simulink library "mylib"  (R2020a)
settings: Solver=VariableStepAuto  StartTime=0.0  StopTime=10.0  RelTol=1e-3
undefined symbols (not defined in the file): d_du_max_pu, dir_to_bus1, dir_to_bus_0L, dir_to_bus_2, dir_to_line1, dir_to_line_0L, dir_to_line_2, du_max_pu, du_ph_max_pu, Fi_0, Fi_T_H, Fi_T_L, Fi_T_M, I0_calc_0L, I0_comp_H, I0_comp_L, I0_comp_M, I0_max_0L, I2_max_2, I_diff1, I_diff2, I_diff3, I_diff4, I_diff5, I_diff_to, I_hight_CT1_G, I_hight_CT2_G, I_low_CT1, I_low_CT2, I_max1, I_max2, I_max3, I_max4, I_max5, I_min_sec_CT1, I_min_sec_CT2, I_unb, Iph_max_0L, Iph_max_2, jmp_in_zone, jmp_in_zone_0L, jmp_in_zone_2, K_dop, max_min1, only_K1_0L, only_K1_2, only_K2_0L, only_K2_2, only_K3_0L, only_K3_2, P_ctl_0, PQ_Fi_ctl_0, Q_ctl_0, S_set_0, set, set1, T_fast, T_I_ctl, T_off, T_on ... (+15)
libraries: $bdroot x184, powerlib_meascontrol x97
(part 13 of 14)

== system mylib/Inverse time-delay/IEC Inverse time-delay/Equation IEC/Zero_check ==
  in : Inport
  Constant : Constant  Value=0
  Constant1 : Constant  Value=0.000001
  Relational Operator : RelationalOperator  Operator===  OutDataTypeStr=boolean  RndMeth=Simplest
  Switch : Switch  Criteria=u2 > Threshold
  out : Outport
  wires:
  in/1 -> Switch/3, Relational Operator/1
  Constant/1 -> Relational Operator/2
  Relational Operator/1 -> Switch/2
  Constant1/1 -> Switch/1
  Switch/1 -> out/1

== system mylib/Inverse time-delay/IEC Inverse time-delay/Equation IEC/Zero_check1 ==
  in : Inport
  Constant : Constant  Value=0
  Constant1 : Constant  Value=0.000001
  Relational Operator : RelationalOperator  Operator===  OutDataTypeStr=boolean  RndMeth=Simplest
  Switch : Switch  Criteria=u2 > Threshold
  out : Outport
  wires:
  in/1 -> Switch/3, Relational Operator/1
  Constant/1 -> Relational Operator/2
  Relational Operator/1 -> Switch/2
  Constant1/1 -> Switch/1
  Switch/1 -> out/1

== system mylib/Inverse time-delay/IEC Inverse time-delay inductive disk relay/Equation IEC_idr/Zero_check ==
  in : Inport
  Constant : Constant  Value=0
  Constant1 : Constant  Value=0.000001
  Relational Operator : RelationalOperator  Operator===  OutDataTypeStr=boolean  RndMeth=Simplest
  Switch : Switch  Criteria=u2 > Threshold
  out : Outport
  wires:
  in/1 -> Switch/3, Relational Operator/1
  Constant/1 -> Relational Operator/2
  Relational Operator/1 -> Switch/2
  Constant1/1 -> Switch/1
  Switch/1 -> out/1

== system mylib/Inverse time-delay/IEC Inverse time-delay inductive disk relay/Equation IEC_idr/Zero_check1 ==
  in : Inport
  Constant : Constant  Value=0
  Constant1 : Constant  Value=0.000001
  Relational Operator : RelationalOperator  Operator===  OutDataTypeStr=boolean  RndMeth=Simplest
  Switch : Switch  Criteria=u2 > Threshold
  out : Outport
  wires:
  in/1 -> Switch/3, Relational Operator/1
  Constant/1 -> Relational Operator/2
  Relational Operator/1 -> Switch/2
  Constant1/1 -> Switch/1
  Switch/1 -> out/1

== system mylib/st_inverse/Inverse time-delay/ANSI Inverse time-delay/Equation ANSI ==
  B : Inport
  I : Inport  Port=2
  Ip : Inport  Port=3
  A : Inport  Port=4
  C : Inport  Port=5
  D : Inport  Port=6
  Add : Sum  Inputs=+-
  Add1 : Sum
  Constant18 : Constant  Value=20
  Constant3 : Constant
  Divide : Product  Inputs=*/
  Divide1 : Product  Inputs=*/
  Divide3 : Product  Inputs=**
  Math Function : Math  Operator=pow  SaturateOnIntegerOverflow=on
  Relational Operator : RelationalOperator  OutDataTypeStr=boolean  RndMeth=Simplest
  Switch : Switch  Criteria=u2 > Threshold
  Zero_check : Subsystem
  Zero_check1 : Subsystem
  td : Outport
  wires:
  I/1 -> Divide/1
  B/1 -> Divide1/1
  D/1 -> Divide3/2
  Divide3/1 -> td/1
  Ip/1 -> Zero_check/1(in)
  Zero_check/1(out) -> Divide/2
  Add/1 -> Zero_check1/1(in)
  Zero_check1/1(out) -> Divide1/2
  Constant3/1 -> Add/2
  Divide1/1 -> Add1/1
  Add1/1 -> Divide3/1
  C/1 -> Add1/2
  Divide/1 -> Switch/3, Relational Operator/1
  Constant18/1 -> Switch/1, Relational Operator/2
  Relational Operator/1 -> Switch/2
  Switch/1 -> Math Function/1
  A/1 -> Math Function/2
  Math Function/1 -> Add/1

== system mylib/st_inverse/Inverse time-delay/ANSI Inverse time-delay/Сoefficient_1 ==
  A_in : Inport
  B_in : Inport  Port=2
  C_in : Inport  Port=3
  N : Inport  Port=4
  Constant1 : Constant  Value=0.17966
  Constant3 : Constant  Value=2.0938
  Constant6 : Constant  Value=8.9341
  Switch : Switch  Criteria=u2 > Threshold
  Switch1 : Switch  Criteria=u2 > Threshold
  Switch2 : Switch  Criteria=u2 > Threshold
  A_out : Outport
  B_out : Outport  Port=2
  C_out : Outport  Port=3
  wires:
  Switch1/1 -> B_out/1
  Constant3/1 -> Switch/1
  Constant6/1 -> Switch1/1
  Switch/1 -> A_out/1
  N/1 -> Switch2/2, Switch/2, Switch1/2
  A_in/1 -> Switch/3
  B_in/1 -> Switch1/3
  C_in/1 -> Switch2/3
  Constant1/1 -> Switch2/1
  Switch2/1 -> C_out/1

== system mylib/st_inverse/Inverse time-delay/ANSI Inverse time-delay/Сoefficient_2 ==
  A_in : Inport
  B_in : Inport  Port=2
  C_in : Inport  Port=3
  N : Inport  Port=4
  Constant1 : Constant  Value=0.03393
  Constant3 : Constant  Value=1.2969
  Constant6 : Constant  Value=0.2663
  Switch : Switch  Criteria=u2 > Threshold
  Switch1 : Switch  Criteria=u2 > Threshold
  Switch2 : Switch  Criteria=u2 > Threshold
  A_out : Outport
  B_out : Outport  Port=2
  C_out : Outport  Port=3
  wires:
  Switch1/1 -> B_out/1
  Constant3/1 -> Switch/1
  Constant6/1 -> Switch1/1
  Switch/1 -> A_out/1
  N/1 -> Switch2/2, Switch/2, Switch1/2
  A_in/1 -> Switch/3
  B_in/1 -> Switch1/3
  C_in/1 -> Switch2/3
  Constant1/1 -> Switch2/1
  Switch2/1 -> C_out/1

== system mylib/st_inverse/Inverse time-delay/ANSI Inverse time-delay/Сoefficient_3 ==
  A_in : Inport
  B_in : Inport  Port=2
  C_in : Inport  Port=3
  N : Inport  Port=4
  Constant1 : Constant  Value=2.18592
  Constant3 : Constant
  Constant6 : Constant  Value=5.6143
  Switch : Switch  Criteria=u2 > Threshold
  Switch1 : Switch  Criteria=u2 > Threshold
  Switch2 : Switch  Criteria=u2 > Threshold
  A_out : Outport
  B_out : Outport  Port=2
  C_out : Outport  Port=3
  wires:
  Switch1/1 -> B_out/1
  Constant3/1 -> Switch/1
  Constant6/1 -> Switch1/1
  Switch/1 -> A_out/1
  N/1 -> Switch2/2, Switch/2, Switch1/2
  A_in/1 -> Switch/3
  B_in/1 -> Switch1/3
  C_in/1 -> Switch2/3
  Constant1/1 -> Switch2/1
  Switch2/1 -> C_out/1

== system mylib/st_inverse/Inverse time-delay/ANSI Inverse time-delay/Сoefficient_4 ==
  A_in : Inport
  B_in : Inport  Port=2
  C_in : Inport  Port=3
  N : Inport  Port=4
  Constant1 : Constant  Value=0.0228
  Constant3 : Constant  Value=0.02
  Constant6 : Constant  Value=0.0103
  Switch : Switch  Criteria=u2 > Threshold
  Switch1 : Switch  Criteria=u2 > Threshold
  Switch2 : Switch  Criteria=u2 > Threshold
  A_out : Outport
  B_out : Outport  Port=2
  C_out : Outport  Port=3
  wires:
  Switch1/1 -> B_out/1
  Constant3/1 -> Switch/1
  Constant6/1 -> Switch1/1
  Switch/1 -> A_out/1
  N/1 -> Switch2/2, Switch/2, Switch1/2
  A_in/1 -> Switch/3
  B_in/1 -> Switch1/3
  C_in/1 -> Switch2/3
  Constant1/1 -> Switch2/1
  Switch2/1 -> C_out/1

== system mylib/st_inverse/Inverse time-delay/ANSI Inverse time-delay/Сoefficient_5 ==
  A_in : Inport
  B_in : Inport  Port=2
  C_in : Inport  Port=3
  N : Inport  Port=4
  Constant1 : Constant  Value=0.0982
  Constant3 : Constant  Value=2
  Constant6 : Constant  Value=3.922
  Switch : Switch  Criteria=u2 > Threshold
  Switch1 : Switch  Criteria=u2 > Threshold
  Switch2 : Switch  Criteria=u2 > Threshold
  A_out : Outport
  B_out : Outport  Port=2
  C_out : Outport  Port=3
  wires:
  Switch1/1 -> B_out/1
  Constant3/1 -> Switch/1
  Constant6/1 -> Switch1/1
  Switch/1 -> A_out/1
  N/1 -> Switch2/2, Switch/2, Switch1/2
  A_in/1 -> Switch/3
  B_in/1 -> Switch1/3
  C_in/1 -> Switch2/3
  Constant1/1 -> Switch2/1
  Switch2/1 -> C_out/1

== system mylib/st_inverse/Inverse time-delay/ANSI Inverse time-delay/Сoefficient_6 ==
  A_in : Inport
  B_in : Inport  Port=2
  C_in : Inport  Port=3
  N : Inport  Port=4
  Constant1 : Constant  Value=0.02434
  Constant3 : Constant  Value=2
  Constant6 : Constant  Value=5.64
  Switch : Switch  Criteria=u2 > Threshold
  Switch1 : Switch  Criteria=u2 > Threshold
  Switch2 : Switch  Criteria=u2 > Threshold
  A_out : Outport
  B_out : Outport  Port=2
  C_out : Outport  Port=3
  wires:
  Switch1/1 -> B_out/1
  Constant3/1 -> Switch/1
  Constant6/1 -> Switch1/1
  Switch/1 -> A_out/1
  N/1 -> Switch2/2, Switch/2, Switch1/2
  A_in/1 -> Switch/3
  B_in/1 -> Switch1/3
  C_in/1 -> Switch2/3
  Constant1/1 -> Switch2/1
  Switch2/1 -> C_out/1

== system mylib/st_inverse/Inverse time-delay/ANSI Inverse time-delay/Сoefficient_7 ==
  A_in : Inport
  B_in : Inport  Port=2
  C_in : Inport  Port=3
  N : Inport  Port=4
  Constant1 : Constant  Value=0.21359
  Constant3 : Constant  Value=1.5825
  Constant6 : Constant  Value=0.4797
  Switch : Switch  Criteria=u2 > Threshold
  Switch1 : Switch  Criteria=u2 > Threshold
  Switch2 : Switch  Criteria=u2 > Threshold
  A_out : Outport
  B_out : Outport  Port=2
  C_out : Outport  Port=3
  wires:
  Switch1/1 -> B_out/1
  Constant3/1 -> Switch/1
  Constant6/1 -> Switch1/1
  Switch/1 -> A_out/1
  N/1 -> Switch2/2, Switch/2, Switch1/2
  A_in/1 -> Switch/3
  B_in/1 -> Switch1/3
  C_in/1 -> Switch2/3
  Constant1/1 -> Switch2/1
  Switch2/1 -> C_out/1

== system mylib/st_inverse/Inverse time-delay/ANSI Inverse time-delay/Сoefficient_8 User ==
  A_in : Inport
  B_in : Inport  Port=2
  C_in : Inport  Port=3
  N : Inport  Port=4
  Au : Inport  Port=5
  Bu : Inport  Port=6
  Cu : Inport  Port=7
  Switch : Switch  Criteria=u2 > Threshold
  Switch1 : Switch  Criteria=u2 > Threshold
  Switch2 : Switch  Criteria=u2 > Threshold
  B_out : Outport
  A_out : Outport  Port=2
  C_out : Outport  Port=3
  wires:
  Switch1/1 -> B_out/1
  Au/1 -> Switch/1
  Bu/1 -> Switch1/1
  Switch/1 -> A_out/1
  N/1 -> Switch2/2, Switch/2, Switch1/2
  A_in/1 -> Switch/3
  B_in/1 -> Switch1/3
  C_in/1 -> Switch2/3
  Cu/1 -> Switch2/1
  Switch2/1 -> C_out/1

== system mylib/st_inverse/Inverse time-delay/ANSI Inverse time-delay inductive disk relay/Equation ANSI_idr ==
  B : Inport
  I : Inport  Port=2
  Ip : Inport  Port=3
  A : Inport  Port=4
  C : Inport  Port=5
  D : Inport  Port=6
  Add : Sum  Inputs=+-
  Add1 : Sum
  Constant3 : Constant
  Divide : Product  Inputs=*/
  Divide1 : Product  Inputs=*/
  Divide3 : Product  Inputs=**
  Math Function : Math  Operator=pow  SaturateOnIntegerOverflow=on
  Zero_check : Subsystem
  Zero_check1 : Subsystem
  td : Outport
  wires:
  I/1 -> Divide/1
  B/1 -> Divide1/1
  D/1 -> Divide3/2
  Divide3/1 -> td/1
  Divide/1 -> Math Function/1
  A/1 -> Math Function/2
  Ip/1 -> Zero_check/1(in)
  Zero_check/1(out) -> Divide/2
  Add/1 -> Zero_check1/1(in)
  Zero_check1/1(out) -> Divide1/2
  Constant3/1 -> Add/1
  Divide1/1 -> Add1/1
  Add1/1 -> Divide3/1
  C/1 -> Add1/2
  Math Function/1 -> Add/2

== system mylib/st_inverse/Inverse time-delay/ANSI Inverse time-delay inductive disk relay/Сoefficient_1 ==
  A_in : Inport
  B_in : Inport  Port=2
  C_in : Inport  Port=3
  N : Inport  Port=4
  Constant1 : Constant  Value=0
  Constant3 : Constant  Value=2.0938
  Constant6 : Constant  Value=8.8
  Switch : Switch  Criteria=u2 > Threshold
  Switch1 : Switch  Criteria=u2 > Threshold
  Switch2 : Switch  Criteria=u2 > Threshold
  A_out : Outport
  B_out : Outport  Port=2
  C_out : Outport  Port=3
  wires:
  Switch1/1 -> B_out/1
  Constant3/1 -> Switch/1
  Constant6/1 -> Switch1/1
  Switch/1 -> A_out/1
  N/1 -> Switch2/2, Switch/2, Switch1/2
  A_in/1 -> Switch/3
  B_in/1 -> Switch1/3
  C_in/1 -> Switch2/3
  Constant1/1 -> Switch2/1
  Switch2/1 -> C_out/1

== system mylib/st_inverse/Inverse time-delay/ANSI Inverse time-delay inductive disk relay/Сoefficient_2 ==
  A_in : Inport
  B_in : Inport  Port=2
  C_in : Inport  Port=3
  N : Inport  Port=4
  Constant1 : Constant  Value=0
  Constant3 : Constant  Value=1.2969
  Constant6 : Constant  Value=0.831
  Switch : Switch  Criteria=u2 > Threshold
  Switch1 : Switch  Criteria=u2 > Threshold
  Switch2 : Switch  Criteria=u2 > Threshold
  A_out : Outport
  B_out : Outport  Port=2
  C_out : Outport  Port=3
  wires:
  Switch1/1 -> B_out/1
  Constant3/1 -> Switch/1
  Constant6/1 -> Switch1/1
  Switch/1 -> A_out/1
  N/1 -> Switch2/2, Switch/2, Switch1/2
  A_in/1 -> Switch/3
  B_in/1 -> Switch1/3
  C_in/1 -> Switch2/3
  Constant1/1 -> Switch2/1
  Switch2/1 -> C_out/1

== system mylib/st_inverse/Inverse time-delay/ANSI Inverse time-delay inductive disk relay/Сoefficient_3 ==
  A_in : Inport
  B_in : Inport  Port=2
  C_in : Inport  Port=3
  N : Inport  Port=4
  Constant1 : Constant  Value=0
  Constant3 : Constant
  Constant6 : Constant  Value=12.9
  Switch : Switch  Criteria=u2 > Threshold
  Switch1 : Switch  Criteria=u2 > Threshold
  Switch2 : Switch  Criteria=u2 > Threshold
  A_out : Outport
  B_out : Outport  Port=2
  C_out : Outport  Port=3
  wires:
  Switch1/1 -> B_out/1
  Constant3/1 -> Switch/1
  Constant6/1 -> Switch1/1
  Switch/1 -> A_out/1
  N/1 -> Switch2/2, Switch/2, Switch1/2
  A_in/1 -> Switch/3
  B_in/1 -> Switch1/3
  C_in/1 -> Switch2/3
  Constant1/1 -> Switch2/1
  Switch2/1 -> C_out/1

== system mylib/st_inverse/Inverse time-delay/ANSI Inverse time-delay inductive disk relay/Сoefficient_4 ==
  A_in : Inport
  B_in : Inport  Port=2
  C_in : Inport  Port=3
  N : Inport  Port=4
  Constant1 : Constant  Value=0
  Constant3 : Constant  Value=2
  Constant6 : Constant  Value=0.97
  Switch : Switch  Criteria=u2 > Threshold
  Switch1 : Switch  Criteria=u2 > Threshold
  Switch2 : Switch  Criteria=u2 > Threshold
  A_out : Outport
  B_out : Outport  Port=2
  C_out : Outport  Port=3
  wires:
  Switch1/1 -> B_out/1
  Constant3/1 -> Switch/1
  Constant6/1 -> Switch1/1
  Switch/1 -> A_out/1
  N/1 -> Switch2/2, Switch/2, Switch1/2
  A_in/1 -> Switch/3
  B_in/1 -> Switch1/3
  C_in/1 -> Switch2/3
  Constant1/1 -> Switch2/1
  Switch2/1 -> C_out/1

== system mylib/st_inverse/Inverse time-delay/ANSI Inverse time-delay inductive disk relay/Сoefficient_5 ==
  A_in : Inport
  B_in : Inport  Port=2
  C_in : Inport  Port=3
  N : Inport  Port=4
  Constant1 : Constant  Value=0
  Constant3 : Constant  Value=2
  Constant6 : Constant  Value=4.32
  Switch : Switch  Criteria=u2 > Threshold
  Switch1 : Switch  Criteria=u2 > Threshold
  Switch2 : Switch  Criteria=u2 > Threshold
  A_out : Outport
  B_out : Outport  Port=2
  C_out : Outport  Port=3
  wires:
  Switch1/1 -> B_out/1
  Constant3/1 -> Switch/1
  Constant6/1 -> Switch1/1
  Switch/1 -> A_out/1
  N/1 -> Switch2/2, Switch/2, Switch1/2
  A_in/1 -> Switch/3
  B_in/1 -> Switch1/3
  C_in/1 -> Switch2/3
  Constant1/1 -> Switch2/1
  Switch2/1 -> C_out/1

== system mylib/st_inverse/Inverse time-delay/ANSI Inverse time-delay inductive disk relay/Сoefficient_6 ==
  A_in : Inport
  B_in : Inport  Port=2
  C_in : Inport  Port=3
  N : Inport  Port=4
  Constant1 : Constant  Value=0
  Constant3 : Constant  Value=2
  Constant6 : Constant  Value=5.82
  Switch : Switch  Criteria=u2 > Threshold
  Switch1 : Switch  Criteria=u2 > Threshold
  Switch2 : Switch  Criteria=u2 > Threshold
  A_out : Outport
  B_out : Outport  Port=2
  C_out : Outport  Port=3
  wires:
  Switch1/1 -> B_out/1
  Constant3/1 -> Switch/1
  Constant6/1 -> Switch1/1
  Switch/1 -> A_out/1
  N/1 -> Switch2/2, Switch/2, Switch1/2
  A_in/1 -> Switch/3
  B_in/1 -> Switch1/3
  C_in/1 -> Switch2/3
  Constant1/1 -> Switch2/1
  Switch2/1 -> C_out/1

== system mylib/st_inverse/Inverse time-delay/ANSI Inverse time-delay inductive disk relay/Сoefficient_7 ==
  A_in : Inport
  B_in : Inport  Port=2
  C_in : Inport  Port=3
  N : Inport  Port=4
  Constant1 : Constant  Value=0.21359
  Constant3 : Constant  Value=1.5625
  Constant6 : Constant  Value=1.0394
  Switch : Switch  Criteria=u2 > Threshold
  Switch1 : Switch  Criteria=u2 > Threshold
  Switch2 : Switch  Criteria=u2 > Threshold
  A_out : Outport
  B_out : Outport  Port=2
  C_out : Outport  Port=3
  wires:
  Switch1/1 -> B_out/1
  Constant3/1 -> Switch/1
  Constant6/1 -> Switch1/1
  Switch/1 -> A_out/1
  N/1 -> Switch2/2, Switch/2, Switch1/2
  A_in/1 -> Switch/3
  B_in/1 -> Switch1/3
  C_in/1 -> Switch2/3
  Constant1/1 -> Switch2/1
  Switch2/1 -> C_out/1

== system mylib/st_inverse/Inverse time-delay/ANSI Inverse time-delay inductive disk relay/Сoefficient_8 User ==
  A_in : Inport
  B_in : Inport  Port=2
  C_in : Inport  Port=3
  N : Inport  Port=4
  Au : Inport  Port=5
  Bu : Inport  Port=6
  Cu : Inport  Port=7
  Switch : Switch  Criteria=u2 > Threshold
  Switch1 : Switch  Criteria=u2 > Threshold
  Switch2 : Switch  Criteria=u2 > Threshold
  B_out : Outport
  A_out : Outport  Port=2
  C_out : Outport  Port=3
  wires:
  Switch1/1 -> B_out/1
  Au/1 -> Switch/1
  Bu/1 -> Switch1/1
  Switch/1 -> A_out/1
  N/1 -> Switch2/2, Switch/2, Switch1/2
  A_in/1 -> Switch/3
  B_in/1 -> Switch1/3
  C_in/1 -> Switch2/3
  Cu/1 -> Switch2/1
  Switch2/1 -> C_out/1

== system mylib/st_inverse/Inverse time-delay/IEC Inverse time-delay/Equation IEC ==
  k : Inport
  I : Inport  Port=2
  a : Inport  Port=3
  Ip : Inport  Port=4
  Tb : Inport  Port=5
  Add : Sum  Inputs=+-
  Constant18 : Constant  Value=20
  Constant3 : Constant
  Divide : Product  Inputs=*/
  Divide1 : Product  Inputs=*/
  Divide2 : Product  Inputs=*/
  Divide3 : Product  Inputs=**
  Math Function : Math  Operator=pow  SaturateOnIntegerOverflow=on
  Relational Operator : RelationalOperator  OutDataTypeStr=boolean  RndMeth=Simplest
  Switch : Switch  Criteria=u2 > Threshold
  Zero_check : Subsystem
  Zero_check1 : Subsystem
  td : Outport
  wires:
  I/1 -> Divide/1, Divide2/1
  Math Function/1 -> Add/1
  Constant3/1 -> Add/2
  k/1 -> Divide1/1
  Divide1/1 -> Divide3/1
  Tb/1 -> Divide3/2
  Divide3/1 -> td/1
  a/1 -> Math Function/2
  Ip/1 -> Zero_check/1(in)
  Zero_check/1(out) -> Divide2/2, Divide/2
  Add/1 -> Zero_check1/1(in)
  Zero_check1/1(out) -> Divide1/2
  Divide2/1 -> Relational Operator/1
  Constant18/1 -> Switch/1, Relational Operator/2
  Relational Operator/1 -> Switch/2
  Divide/1 -> Switch/3
  Switch/1 -> Math Function/1

== system mylib/st_inverse/Inverse time-delay/IEC Inverse time-delay/Сoefficient_1 ==
  k_in : Inport
  a_in : Inport  Port=2
  N : Inport  Port=3
  Constant3 : Constant  Value=0.14
  Constant6 : Constant  Value=0.02
  Switch : Switch  Criteria=u2 > Threshold
  Switch1 : Switch  Criteria=u2 > Threshold
  k_out : Outport
  a_out : Outport  Port=2
  wires:
  Switch1/1 -> a_out/1
  Constant3/1 -> Switch/1
  Constant6/1 -> Switch1/1
  Switch/1 -> k_out/1
  N/1 -> Switch/2, Switch1/2
  k_in/1 -> Switch/3
  a_in/1 -> Switch1/3

== system mylib/st_inverse/Inverse time-delay/IEC Inverse time-delay/Сoefficient_2 ==
  k_in : Inport
  a_in : Inport  Port=2
  N : Inport  Port=3
  Constant3 : Constant  Value=13.5
  Constant6 : Constant
  Switch : Switch  Criteria=u2 > Threshold
  Switch1 : Switch  Criteria=u2 > Threshold
  k_out : Outport
  a_out : Outport  Port=2
  wires:
  Switch1/1 -> a_out/1
  Constant3/1 -> Switch/1
  Constant6/1 -> Switch1/1
  Switch/1 -> k_out/1
  N/1 -> Switch/2, Switch1/2
  k_in/1 -> Switch/3
  a_in/1 -> Switch1/3

== system mylib/st_inverse/Inverse time-delay/IEC Inverse time-delay/Сoefficient_3 ==
  k_in : Inport
  a_in : Inport  Port=2
  N : Inport  Port=3
  Constant3 : Constant  Value=120
  Constant6 : Constant
  Switch : Switch  Criteria=u2 > Threshold
  Switch1 : Switch  Criteria=u2 > Threshold
  k_out : Outport
  a_out : Outport  Port=2
  wires:
  Switch1/1 -> a_out/1
  Constant3/1 -> Switch/1
  Constant6/1 -> Switch1/1
  Switch/1 -> k_out/1
  N/1 -> Switch/2, Switch1/2
  k_in/1 -> Switch/3
  a_in/1 -> Switch1/3

== system mylib/st_inverse/Inverse time-delay/IEC Inverse time-delay/Сoefficient_4 ==
  k_in : Inport
  a_in : Inport  Port=2
  N : Inport  Port=3
  Constant3 : Constant  Value=80
  Constant6 : Constant  Value=2
  Switch : Switch  Criteria=u2 > Threshold
  Switch1 : Switch  Criteria=u2 > Threshold
  k_out : Outport
  a_out : Outport  Port=2
  wires:
  Switch1/1 -> a_out/1
  Constant3/1 -> Switch/1
  Constant6/1 -> Switch1/1
  Switch/1 -> k_out/1
  N/1 -> Switch/2, Switch1/2
  k_in/1 -> Switch/3
  a_in/1 -> Switch1/3

== system mylib/st_inverse/Inverse time-delay/IEC Inverse time-delay/Сoefficient_5 User ==
  k : Inport
  a : Inport  Port=2
  N : Inport  Port=3
  k_u : Inport  Port=4
  a_u : Inport  Port=5
  Switch : Switch  Criteria=u2 > Threshold
  Switch1 : Switch  Criteria=u2 > Threshold
  k_out : Outport
  a_out : Outport  Port=2
  wires:
  Switch1/1 -> a_out/1
  k_u/1 -> Switch/1
  a_u/1 -> Switch1/1
  Switch/1 -> k_out/1
  N/1 -> Switch/2, Switch1/2
  k/1 -> Switch/3
  a/1 -> Switch1/3

== system mylib/st_inverse/Inverse time-delay/IEC Inverse time-delay inductive disk relay/Equation IEC_idr ==
  k : Inport
  I : Inport  Port=2
  a : Inport  Port=3
  Ip : Inport  Port=4
  Tb : Inport  Port=5
  Add : Sum  Inputs=+-
  Constant3 : Constant
  Divide : Product  Inputs=*/
  Divide1 : Product  Inputs=*/
  Divide3 : Product  Inputs=**
  Math Function : Math  Operator=pow  SaturateOnIntegerOverflow=on
  Zero_check : Subsystem
  Zero_check1 : Subsystem
  td : Outport
  wires:
  I/1 -> Divide/1
  k/1 -> Divide1/1
  Divide1/1 -> Divide3/1
  Tb/1 -> Divide3/2
  Divide3/1 -> td/1
  Divide/1 -> Math Function/1
  a/1 -> Math Function/2
  Ip/1 -> Zero_check/1(in)
  Zero_check/1(out) -> Divide/2
  Add/1 -> Zero_check1/1(in)
  Zero_check1/1(out) -> Divide1/2
  Math Function/1 -> Add/2
  Constant3/1 -> Add/1

== system mylib/st_inverse/Inverse time-delay/IEC Inverse time-delay inductive disk relay/Сoefficient_1 ==
  k_in : Inport
  a_in : Inport  Port=2
  N : Inport  Port=3
  Constant3 : Constant  Value=9.7
  Constant6 : Constant  Value=2
  Switch : Switch  Criteria=u2 > Threshold
  Switch1 : Switch  Criteria=u2 > Threshold
  k_out : Outport
  a_out : Outport  Port=2
  wires:
  Switch1/1 -> a_out/1
  Constant3/1 -> Switch/1
  Constant6/1 -> Switch1/1
  Switch/1 -> k_out/1
  N/1 -> Switch/2, Switch1/2
  k_in/1 -> Switch/3
  a_in/1 -> Switch1/3

== system mylib/st_inverse/Inverse time-delay/IEC Inverse time-delay inductive disk relay/Сoefficient_2 ==
  k_in : Inport
  a_in : Inport  Port=2
  N : Inport  Port=3
  Constant3 : Constant  Value=43.2
  Constant6 : Constant  Value=2
  Switch : Switch  Criteria=u2 > Threshold
  Switch1 : Switch  Criteria=u2 > Threshold
  k_out : Outport
  a_out : Outport  Port=2
  wires:
  Switch1/1 -> a_out/1
  Constant3/1 -> Switch/1
  Constant6/1 -> Switch1/1
  Switch/1 -> k_out/1
  N/1 -> Switch/2, Switch1/2
  k_in/1 -> Switch/3
  a_in/1 -> Switch1/3

== system mylib/st_inverse/Inverse time-delay/IEC Inverse time-delay inductive disk relay/Сoefficient_3 ==
  k_in : Inport
  a_in : Inport  Port=2
  N : Inport  Port=3
  Constant3 : Constant  Value=58.2
  Constant6 : Constant  Value=2
  Switch : Switch  Criteria=u2 > Threshold
  Switch1 : Switch  Criteria=u2 > Threshold
  k_out : Outport
  a_out : Outport  Port=2
  wires:
  Switch1/1 -> a_out/1
  Constant3/1 -> Switch/1
  Constant6/1 -> Switch1/1
  Switch/1 -> k_out/1
  N/1 -> Switch/2, Switch1/2
  k_in/1 -> Switch/3
  a_in/1 -> Switch1/3

== system mylib/st_inverse/Inverse time-delay/IEC Inverse time-delay inductive disk relay/Сoefficient_4 ==
  k_in : Inport
  a_in : Inport  Port=2
  N : Inport  Port=3
  Constant3 : Constant  Value=80
  Constant6 : Constant  Value=2
  Switch : Switch  Criteria=u2 > Threshold
  Switch1 : Switch  Criteria=u2 > Threshold
  k_out : Outport
  a_out : Outport  Port=2
  wires:
  Switch1/1 -> a_out/1
  Constant3/1 -> Switch/1
  Constant6/1 -> Switch1/1
  Switch/1 -> k_out/1
  N/1 -> Switch/2, Switch1/2
  k_in/1 -> Switch/3
  a_in/1 -> Switch1/3

== system mylib/st_inverse/Inverse time-delay/IEC Inverse time-delay inductive disk relay/Сoefficient_5 User ==
  k : Inport
  a : Inport  Port=2
  N : Inport  Port=3
  k_u : Inport  Port=4
  a_u : Inport  Port=5
  Switch : Switch  Criteria=u2 > Threshold
  Switch1 : Switch  Criteria=u2 > Threshold
  k_out : Outport
  a_out : Outport  Port=2
  wires:
  Switch1/1 -> a_out/1
  k_u/1 -> Switch/1
  a_u/1 -> Switch1/1
  Switch/1 -> k_out/1
  N/1 -> Switch/2, Switch1/2
  k/1 -> Switch/3
  a/1 -> Switch1/3

== system mylib/278_dzt_v1/diff_brake/calc_brake_Ia/cut_brake_1/ADD_B ==
  Y1 : Inport
  X2 : Inport  Port=2
  Y2 : Inport  Port=3
  X1 : Inport  Port=4
  1 : Product
  2 : Sum  Inputs=+-
  3 : Product  Inputs=*/  RndMeth=Zero  SaturateOnIntegerOverflow=on
  4 : Product
  5 : Sum  Inputs=+-
  out : Outport
  wires:
  3/1 -> out/1
  4/1 -> 5/2
  Y2/1 -> 4/1
  2/1 -> 3/2
  5/1 -> 3/1
  1/1 -> 5/1
  X2/1 -> 2/1, 1/2
  X1/1 -> 4/2, 2/2
  Y1/1 -> 1/1

== system mylib/278_dzt_v1/diff_brake/calc_brake_Ia/cut_brake_1/ADD_K ==
  Y2 : Inport
  Y1 : Inport  Port=2
  X2 : Inport  Port=3
  X1 : Inport  Port=4
  1 : Sum  Inputs=+-
  2 : Sum  Inputs=+-
  3 : Product  Inputs=*/  RndMeth=Zero  SaturateOnIntegerOverflow=on
  out : Outport
  wires:
  Y1/1 -> 1/2
  Y2/1 -> 1/1
  X1/1 -> 2/2
  X2/1 -> 2/1
  3/1 -> out/1
  2/1 -> 3/2
  1/1 -> 3/1

== system mylib/278_dzt_v1/diff_brake/calc_brake_Ia/cut_brake_1/z_ch ==
  in1 : Inport
  in2 : Inport  Port=2
  1 : RelationalOperator  Operator===  OutDataTypeStr=boolean  RndMeth=Simplest
  2 : RelationalOperator  Operator===  OutDataTypeStr=boolean  RndMeth=Simplest
  3 : Logic  AllPortsSameDT=off  OutDataTypeStr=boolean
  36 : Constant  Value=0
  out : Outport
  wires:
  3/1 -> out/1
  2/1 -> 3/2
  1/1 -> 3/1
  36/1 -> 2/2, 1/2
  in2/1 -> 2/1
  in1/1 -> 1/1

== system mylib/278_dzt_v1/diff_brake/calc_brake_Ia/cut_brake_1/z_ch1 ==
  in1 : Inport
  in2 : Inport  Port=2
  1 : RelationalOperator  Operator===  OutDataTypeStr=boolean  RndMeth=Simplest
  2 : RelationalOperator  Operator===  OutDataTypeStr=boolean  RndMeth=Simplest
  3 : Logic  AllPortsSameDT=off  OutDataTypeStr=boolean
  36 : Constant  Value=0
  out : Outport
  wires:
  3/1 -> out/1
  2/1 -> 3/2
  1/1 -> 3/1
  36/1 -> 2/2, 1/2
  in2/1 -> 2/1
  in1/1 -> 1/1

== system mylib/278_dzt_v1/diff_brake/calc_brake_Ia/cut_brake_1/z_ch2 ==
  in1 : Inport
  in2 : Inport  Port=2
  1 : RelationalOperator  Operator===  OutDataTypeStr=boolean  RndMeth=Simplest
  2 : RelationalOperator  Operator===  OutDataTypeStr=boolean  RndMeth=Simplest
  3 : Logic  AllPortsSameDT=off  OutDataTypeStr=boolean
  36 : Constant  Value=0
  out : Outport
  wires:
  3/1 -> out/1
  2/1 -> 3/2
  1/1 -> 3/1
  36/1 -> 2/2, 1/2
  in2/1 -> 2/1
  in1/1 -> 1/1

== system mylib/278_dzt_v1/diff_brake/calc_brake_Ia/cut_brake_2/ADD_B ==
  Y1 : Inport
  X2 : Inport  Port=2
  Y2 : Inport  Port=3
  X1 : Inport  Port=4
  1 : Product
  2 : Sum  Inputs=+-
  3 : Product  Inputs=*/  RndMeth=Zero  SaturateOnIntegerOverflow=on
  4 : Product
  5 : Sum  Inputs=+-
  out : Outport
  wires:
  3/1 -> out/1
  4/1 -> 5/2
  Y2/1 -> 4/1
  2/1 -> 3/2
  5/1 -> 3/1
  1/1 -> 5/1
  X2/1 -> 2/1, 1/2
  X1/1 -> 4/2, 2/2
  Y1/1 -> 1/1

== system mylib/278_dzt_v1/diff_brake/calc_brake_Ia/cut_brake_2/ADD_K ==
  Y2 : Inport
  Y1 : Inport  Port=2
  X2 : Inport  Port=3
  X1 : Inport  Port=4
  1 : Sum  Inputs=+-
  2 : Sum  Inputs=+-
  3 : Product  Inputs=*/  RndMeth=Zero  SaturateOnIntegerOverflow=on
  out : Outport
  wires:
  Y1/1 -> 1/2
  Y2/1 -> 1/1
  X1/1 -> 2/2
  X2/1 -> 2/1
  3/1 -> out/1
  2/1 -> 3/2
  1/1 -> 3/1

== system mylib/278_dzt_v1/diff_brake/calc_brake_Ia/cut_brake_2/z_ch ==
  in1 : Inport
  in2 : Inport  Port=2
  1 : RelationalOperator  Operator===  OutDataTypeStr=boolean  RndMeth=Simplest
  2 : RelationalOperator  Operator===  OutDataTypeStr=boolean  RndMeth=Simplest
  3 : Logic  AllPortsSameDT=off  OutDataTypeStr=boolean
  36 : Constant  Value=0
  out : Outport
  wires:
  3/1 -> out/1
  2/1 -> 3/2
  1/1 -> 3/1
  36/1 -> 2/2, 1/2
  in2/1 -> 2/1
  in1/1 -> 1/1

== system mylib/278_dzt_v1/diff_brake/calc_brake_Ia/cut_brake_2/z_ch1 ==
  in1 : Inport
  in2 : Inport  Port=2
  1 : RelationalOperator  Operator===  OutDataTypeStr=boolean  RndMeth=Simplest
  2 : RelationalOperator  Operator===  OutDataTypeStr=boolean  RndMeth=Simplest
  3 : Logic  AllPortsSameDT=off  OutDataTypeStr=boolean
  36 : Constant  Value=0
  out : Outport
  wires:
  3/1 -> out/1
  2/1 -> 3/2
  1/1 -> 3/1
  36/1 -> 2/2, 1/2
  in2/1 -> 2/1
  in1/1 -> 1/1

== system mylib/278_dzt_v1/diff_brake/calc_brake_Ia/cut_brake_2/z_ch2 ==
  in1 : Inport
  in2 : Inport  Port=2
  1 : RelationalOperator  Operator===  OutDataTypeStr=boolean  RndMeth=Simplest
  2 : RelationalOperator  Operator===  OutDataTypeStr=boolean  RndMeth=Simplest
  3 : Logic  AllPortsSameDT=off  OutDataTypeStr=boolean
  36 : Constant  Value=0
  out : Outport
  wires:
  3/1 -> out/1
  2/1 -> 3/2
  1/1 -> 3/1
  36/1 -> 2/2, 1/2
  in2/1 -> 2/1
  in1/1 -> 1/1

== system mylib/278_dzt_v1/diff_brake/calc_brake_Ia/cut_brake_3/ADD_B ==
  Y1 : Inport
  X2 : Inport  Port=2
  Y2 : Inport  Port=3
  X1 : Inport  Port=4
  1 : Product
  2 : Sum  Inputs=+-
  3 : Product  Inputs=*/  RndMeth=Zero  SaturateOnIntegerOverflow=on
  4 : Product
  5 : Sum  Inputs=+-
  out : Outport
  wires:
  3/1 -> out/1
  4/1 -> 5/2
  Y2/1 -> 4/1
  2/1 -> 3/2
  5/1 -> 3/1
  1/1 -> 5/1
  X2/1 -> 2/1, 1/2
  X1/1 -> 4/2, 2/2
  Y1/1 -> 1/1

== system mylib/278_dzt_v1/diff_brake/calc_brake_Ia/cut_brake_3/ADD_K ==
  Y2 : Inport
  Y1 : Inport  Port=2
  X2 : Inport  Port=3
  X1 : Inport  Port=4
  1 : Sum  Inputs=+-
  2 : Sum  Inputs=+-
  3 : Product  Inputs=*/  RndMeth=Zero  SaturateOnIntegerOverflow=on
  out : Outport
  wires:
  Y1/1 -> 1/2
  Y2/1 -> 1/1
  X1/1 -> 2/2
  X2/1 -> 2/1
  3/1 -> out/1
  2/1 -> 3/2
  1/1 -> 3/1

== system mylib/278_dzt_v1/diff_brake/calc_brake_Ia/cut_brake_3/z_ch ==
  in1 : Inport
  in2 : Inport  Port=2
  1 : RelationalOperator  Operator===  OutDataTypeStr=boolean  RndMeth=Simplest
  2 : RelationalOperator  Operator===  OutDataTypeStr=boolean  RndMeth=Simplest
  3 : Logic  AllPortsSameDT=off  OutDataTypeStr=boolean
  36 : Constant  Value=0
  out : Outport
  wires:
  3/1 -> out/1
  2/1 -> 3/2
  1/1 -> 3/1
  36/1 -> 2/2, 1/2
  in2/1 -> 2/1
  in1/1 -> 1/1

== system mylib/278_dzt_v1/diff_brake/calc_brake_Ia/cut_brake_3/z_ch1 ==
  in1 : Inport
  in2 : Inport  Port=2
  1 : RelationalOperator  Operator===  OutDataTypeStr=boolean  RndMeth=Simplest
  2 : RelationalOperator  Operator===  OutDataTypeStr=boolean  RndMeth=Simplest
  3 : Logic  AllPortsSameDT=off  OutDataTypeStr=boolean
  36 : Constant  Value=0
  out : Outport
  wires:
  3/1 -> out/1
  2/1 -> 3/2
  1/1 -> 3/1
  36/1 -> 2/2, 1/2
  in2/1 -> 2/1
  in1/1 -> 1/1

== system mylib/278_dzt_v1/diff_brake/calc_brake_Ia/cut_brake_3/z_ch2 ==
  in1 : Inport
  in2 : Inport  Port=2
  1 : RelationalOperator  Operator===  OutDataTypeStr=boolean  RndMeth=Simplest
  2 : RelationalOperator  Operator===  OutDataTypeStr=boolean  RndMeth=Simplest
  3 : Logic  AllPortsSameDT=off  OutDataTypeStr=boolean
  36 : Constant  Value=0
  out : Outport
  wires:
  3/1 -> out/1
  2/1 -> 3/2
  1/1 -> 3/1
  36/1 -> 2/2, 1/2
  in2/1 -> 2/1
  in1/1 -> 1/1

== system mylib/278_dzt_v1/diff_brake/calc_brake_Ia/cut_brake_4/ADD_B ==
  Y1 : Inport
  X2 : Inport  Port=2
  Y2 : Inport  Port=3
  X1 : Inport  Port=4
  1 : Product
  2 : Sum  Inputs=+-
  3 : Product  Inputs=*/  RndMeth=Zero  SaturateOnIntegerOverflow=on
  4 : Product
  5 : Sum  Inputs=+-
  out : Outport
  wires:
  3/1 -> out/1
  4/1 -> 5/2
  Y2/1 -> 4/1
  2/1 -> 3/2
  5/1 -> 3/1
  1/1 -> 5/1
  X2/1 -> 2/1, 1/2
  X1/1 -> 4/2, 2/2
  Y1/1 -> 1/1

== system mylib/278_dzt_v1/diff_brake/calc_brake_Ia/cut_brake_4/ADD_K ==
  Y2 : Inport
  Y1 : Inport  Port=2
  X2 : Inport  Port=3
  X1 : Inport  Port=4
  1 : Sum  Inputs=+-
  2 : Sum  Inputs=+-
  3 : Product  Inputs=*/  RndMeth=Zero  SaturateOnIntegerOverflow=on
  out : Outport
  wires:
  Y1/1 -> 1/2
  Y2/1 -> 1/1
  X1/1 -> 2/2
  X2/1 -> 2/1
  3/1 -> out/1
  2/1 -> 3/2
  1/1 -> 3/1

== system mylib/278_dzt_v1/diff_brake/calc_brake_Ia/cut_brake_4/z_ch ==
  in1 : Inport
  in2 : Inport  Port=2
  1 : RelationalOperator  Operator===  OutDataTypeStr=boolean  RndMeth=Simplest
  2 : RelationalOperator  Operator===  OutDataTypeStr=boolean  RndMeth=Simplest
  3 : Logic  AllPortsSameDT=off  OutDataTypeStr=boolean
  36 : Constant  Value=0
  out : Outport
  wires:
  3/1 -> out/1
  2/1 -> 3/2
  1/1 -> 3/1
  36/1 -> 2/2, 1/2
  in2/1 -> 2/1
  in1/1 -> 1/1

== system mylib/278_dzt_v1/diff_brake/calc_brake_Ia/cut_brake_4/z_ch1 ==
  in1 : Inport
  in2 : Inport  Port=2
  1 : RelationalOperator  Operator===  OutDataTypeStr=boolean  RndMeth=Simplest
  2 : RelationalOperator  Operator===  OutDataTypeStr=boolean  RndMeth=Simplest
  3 : Logic  AllPortsSameDT=off  OutDataTypeStr=boolean
  36 : Constant  Value=0
  out : Outport
  wires:
  3/1 -> out/1
  2/1 -> 3/2
  1/1 -> 3/1
  36/1 -> 2/2, 1/2
  in2/1 -> 2/1
  in1/1 -> 1/1

== system mylib/278_dzt_v1/diff_brake/calc_brake_Ia/cut_brake_4/z_ch2 ==
  in1 : Inport
  in2 : Inport  Port=2
  1 : RelationalOperator  Operator===  OutDataTypeStr=boolean  RndMeth=Simplest
  2 : RelationalOperator  Operator===  OutDataTypeStr=boolean  RndMeth=Simplest
  3 : Logic  AllPortsSameDT=off  OutDataTypeStr=boolean
  36 : Constant  Value=0
  out : Outport
  wires:
  3/1 -> out/1
  2/1 -> 3/2
  1/1 -> 3/1
  36/1 -> 2/2, 1/2
  in2/1 -> 2/1
  in1/1 -> 1/1

== system mylib/278_dzt_v1/diff_brake/calc_brake_Ib/cut_brake_1/ADD_B ==
  Y1 : Inport
  X2 : Inport  Port=2
  Y2 : Inport  Port=3
  X1 : Inport  Port=4
  1 : Product
  2 : Sum  Inputs=+-
  3 : Product  Inputs=*/  RndMeth=Zero  SaturateOnIntegerOverflow=on
  4 : Product
  5 : Sum  Inputs=+-
  out : Outport
  wires:
  3/1 -> out/1
  4/1 -> 5/2
  Y2/1 -> 4/1
  2/1 -> 3/2
  5/1 -> 3/1
  1/1 -> 5/1
  X2/1 -> 2/1, 1/2
  X1/1 -> 4/2, 2/2
  Y1/1 -> 1/1

== system mylib/278_dzt_v1/diff_brake/calc_brake_Ib/cut_brake_1/ADD_K ==
  Y2 : Inport
  Y1 : Inport  Port=2
  X2 : Inport  Port=3
  X1 : Inport  Port=4
  1 : Sum  Inputs=+-
  2 : Sum  Inputs=+-
  3 : Product  Inputs=*/  RndMeth=Zero  SaturateOnIntegerOverflow=on
  out : Outport
  wires:
  Y1/1 -> 1/2
  Y2/1 -> 1/1
  X1/1 -> 2/2
  X2/1 -> 2/1
  3/1 -> out/1
  2/1 -> 3/2
  1/1 -> 3/1

== system mylib/278_dzt_v1/diff_brake/calc_brake_Ib/cut_brake_1/z_ch ==
  in1 : Inport
  in2 : Inport  Port=2
  1 : RelationalOperator  Operator===  OutDataTypeStr=boolean  RndMeth=Simplest
  2 : RelationalOperator  Operator===  OutDataTypeStr=boolean  RndMeth=Simplest
  3 : Logic  AllPortsSameDT=off  OutDataTypeStr=boolean
  36 : Constant  Value=0
  out : Outport
  wires:
  3/1 -> out/1
  2/1 -> 3/2
  1/1 -> 3/1
  36/1 -> 2/2, 1/2
  in2/1 -> 2/1
  in1/1 -> 1/1

== system mylib/278_dzt_v1/diff_brake/calc_brake_Ib/cut_brake_1/z_ch1 ==
  in1 : Inport
  in2 : Inport  Port=2
  1 : RelationalOperator  Operator===  OutDataTypeStr=boolean  RndMeth=Simplest
  2 : RelationalOperator  Operator===  OutDataTypeStr=boolean  RndMeth=Simplest
  3 : Logic  AllPortsSameDT=off  OutDataTypeStr=boolean
  36 : Constant  Value=0
  out : Outport
  wires:
  3/1 -> out/1
  2/1 -> 3/2
  1/1 -> 3/1
  36/1 -> 2/2, 1/2
  in2/1 -> 2/1
  in1/1 -> 1/1

== system mylib/278_dzt_v1/diff_brake/calc_brake_Ib/cut_brake_1/z_ch2 ==
  in1 : Inport
  in2 : Inport  Port=2
  1 : RelationalOperator  Operator===  OutDataTypeStr=boolean  RndMeth=Simplest
  2 : RelationalOperator  Operator===  OutDataTypeStr=boolean  RndMeth=Simplest
  3 : Logic  AllPortsSameDT=off  OutDataTypeStr=boolean
  36 : Constant  Value=0
  out : Outport
  wires:
  3/1 -> out/1
  2/1 -> 3/2
  1/1 -> 3/1
  36/1 -> 2/2, 1/2
  in2/1 -> 2/1
  in1/1 -> 1/1

== system mylib/278_dzt_v1/diff_brake/calc_brake_Ib/cut_brake_2/ADD_B ==
  Y1 : Inport
  X2 : Inport  Port=2
  Y2 : Inport  Port=3
  X1 : Inport  Port=4
  1 : Product
  2 : Sum  Inputs=+-
  3 : Product  Inputs=*/  RndMeth=Zero  SaturateOnIntegerOverflow=on
  4 : Product
  5 : Sum  Inputs=+-
  out : Outport
  wires:
  3/1 -> out/1
  4/1 -> 5/2
  Y2/1 -> 4/1
  2/1 -> 3/2
  5/1 -> 3/1
  1/1 -> 5/1
  X2/1 -> 2/1, 1/2
  X1/1 -> 4/2, 2/2
  Y1/1 -> 1/1

== system mylib/278_dzt_v1/diff_brake/calc_brake_Ib/cut_brake_2/ADD_K ==
  Y2 : Inport
  Y1 : Inport  Port=2
  X2 : Inport  Port=3
  X1 : Inport  Port=4
  1 : Sum  Inputs=+-
  2 : Sum  Inputs=+-
  3 : Product  Inputs=*/  RndMeth=Zero  SaturateOnIntegerOverflow=on
  out : Outport
  wires:
  Y1/1 -> 1/2
  Y2/1 -> 1/1
  X1/1 -> 2/2
  X2/1 -> 2/1
  3/1 -> out/1
  2/1 -> 3/2
  1/1 -> 3/1

== system mylib/278_dzt_v1/diff_brake/calc_brake_Ib/cut_brake_2/z_ch ==
  in1 : Inport
  in2 : Inport  Port=2
  1 : RelationalOperator  Operator===  OutDataTypeStr=boolean  RndMeth=Simplest
  2 : RelationalOperator  Operator===  OutDataTypeStr=boolean  RndMeth=Simplest
  3 : Logic  AllPortsSameDT=off  OutDataTypeStr=boolean
  36 : Constant  Value=0
  out : Outport
  wires:
  3/1 -> out/1
  2/1 -> 3/2
  1/1 -> 3/1
  36/1 -> 2/2, 1/2
  in2/1 -> 2/1
  in1/1 -> 1/1

== system mylib/278_dzt_v1/diff_brake/calc_brake_Ib/cut_brake_2/z_ch1 ==
  in1 : Inport
  in2 : Inport  Port=2
  1 : RelationalOperator  Operator===  OutDataTypeStr=boolean  RndMeth=Simplest
  2 : RelationalOperator  Operator===  OutDataTypeStr=boolean  RndMeth=Simplest
  3 : Logic  AllPortsSameDT=off  OutDataTypeStr=boolean
  36 : Constant  Value=0
  out : Outport
  wires:
  3/1 -> out/1
  2/1 -> 3/2
  1/1 -> 3/1
  36/1 -> 2/2, 1/2
  in2/1 -> 2/1
  in1/1 -> 1/1

== system mylib/278_dzt_v1/diff_brake/calc_brake_Ib/cut_brake_2/z_ch2 ==
  in1 : Inport
  in2 : Inport  Port=2
  1 : RelationalOperator  Operator===  OutDataTypeStr=boolean  RndMeth=Simplest
  2 : RelationalOperator  Operator===  OutDataTypeStr=boolean  RndMeth=Simplest
  3 : Logic  AllPortsSameDT=off  OutDataTypeStr=boolean
  36 : Constant  Value=0
  out : Outport
  wires:
  3/1 -> out/1
  2/1 -> 3/2
  1/1 -> 3/1
  36/1 -> 2/2, 1/2
  in2/1 -> 2/1
  in1/1 -> 1/1

== system mylib/278_dzt_v1/diff_brake/calc_brake_Ib/cut_brake_3/ADD_B ==
  Y1 : Inport
  X2 : Inport  Port=2
  Y2 : Inport  Port=3
  X1 : Inport  Port=4
  1 : Product
  2 : Sum  Inputs=+-
  3 : Product  Inputs=*/  RndMeth=Zero  SaturateOnIntegerOverflow=on
  4 : Product
  5 : Sum  Inputs=+-
  out : Outport
  wires:
  3/1 -> out/1
  4/1 -> 5/2
  Y2/1 -> 4/1
  2/1 -> 3/2
  5/1 -> 3/1
  1/1 -> 5/1
  X2/1 -> 2/1, 1/2
  X1/1 -> 4/2, 2/2
  Y1/1 -> 1/1

== system mylib/278_dzt_v1/diff_brake/calc_brake_Ib/cut_brake_3/ADD_K ==
  Y2 : Inport
  Y1 : Inport  Port=2
  X2 : Inport  Port=3
  X1 : Inport  Port=4
  1 : Sum  Inputs=+-
  2 : Sum  Inputs=+-
  3 : Product  Inputs=*/  RndMeth=Zero  SaturateOnIntegerOverflow=on
  out : Outport
  wires:
  Y1/1 -> 1/2
  Y2/1 -> 1/1
  X1/1 -> 2/2
  X2/1 -> 2/1
  3/1 -> out/1
  2/1 -> 3/2
  1/1 -> 3/1

== system mylib/278_dzt_v1/diff_brake/calc_brake_Ib/cut_brake_3/z_ch ==
  in1 : Inport
  in2 : Inport  Port=2
  1 : RelationalOperator  Operator===  OutDataTypeStr=boolean  RndMeth=Simplest
  2 : RelationalOperator  Operator===  OutDataTypeStr=boolean  RndMeth=Simplest
  3 : Logic  AllPortsSameDT=off  OutDataTypeStr=boolean
  36 : Constant  Value=0
  out : Outport
  wires:
  3/1 -> out/1
  2/1 -> 3/2
  1/1 -> 3/1
  36/1 -> 2/2, 1/2
  in2/1 -> 2/1
  in1/1 -> 1/1

== system mylib/278_dzt_v1/diff_brake/calc_brake_Ib/cut_brake_3/z_ch1 ==
  in1 : Inport
  in2 : Inport  Port=2
  1 : RelationalOperator  Operator===  OutDataTypeStr=boolean  RndMeth=Simplest
  2 : RelationalOperator  Operator===  OutDataTypeStr=boolean  RndMeth=Simplest
  3 : Logic  AllPortsSameDT=off  OutDataTypeStr=boolean
  36 : Constant  Value=0
  out : Outport
  wires:
  3/1 -> out/1
  2/1 -> 3/2
  1/1 -> 3/1
  36/1 -> 2/2, 1/2
  in2/1 -> 2/1
  in1/1 -> 1/1

== system mylib/278_dzt_v1/diff_brake/calc_brake_Ib/cut_brake_3/z_ch2 ==
  in1 : Inport
  in2 : Inport  Port=2
  1 : RelationalOperator  Operator===  OutDataTypeStr=boolean  RndMeth=Simplest
  2 : RelationalOperator  Operator===  OutDataTypeStr=boolean  RndMeth=Simplest
  3 : Logic  AllPortsSameDT=off  OutDataTypeStr=boolean
  36 : Constant  Value=0
  out : Outport
  wires:
  3/1 -> out/1
  2/1 -> 3/2
  1/1 -> 3/1
  36/1 -> 2/2, 1/2
  in2/1 -> 2/1
  in1/1 -> 1/1

== system mylib/278_dzt_v1/diff_brake/calc_brake_Ib/cut_brake_4/ADD_B ==
  Y1 : Inport
  X2 : Inport  Port=2
  Y2 : Inport  Port=3
  X1 : Inport  Port=4
  1 : Product
  2 : Sum  Inputs=+-
  3 : Product  Inputs=*/  RndMeth=Zero  SaturateOnIntegerOverflow=on
  4 : Product
  5 : Sum  Inputs=+-
  out : Outport
  wires:
  3/1 -> out/1
  4/1 -> 5/2
  Y2/1 -> 4/1
  2/1 -> 3/2
  5/1 -> 3/1
  1/1 -> 5/1
  X2/1 -> 2/1, 1/2
  X1/1 -> 4/2, 2/2
  Y1/1 -> 1/1

== system mylib/278_dzt_v1/diff_brake/calc_brake_Ib/cut_brake_4/ADD_K ==
  Y2 : Inport
  Y1 : Inport  Port=2
  X2 : Inport  Port=3
  X1 : Inport  Port=4
  1 : Sum  Inputs=+-
  2 : Sum  Inputs=+-
  3 : Product  Inputs=*/  RndMeth=Zero  SaturateOnIntegerOverflow=on
  out : Outport
  wires:
  Y1/1 -> 1/2
  Y2/1 -> 1/1
  X1/1 -> 2/2
  X2/1 -> 2/1
  3/1 -> out/1
  2/1 -> 3/2
  1/1 -> 3/1

== system mylib/278_dzt_v1/diff_brake/calc_brake_Ib/cut_brake_4/z_ch ==
  in1 : Inport
  in2 : Inport  Port=2
  1 : RelationalOperator  Operator===  OutDataTypeStr=boolean  RndMeth=Simplest
  2 : RelationalOperator  Operator===  OutDataTypeStr=boolean  RndMeth=Simplest
  3 : Logic  AllPortsSameDT=off  OutDataTypeStr=boolean
  36 : Constant  Value=0
  out : Outport
  wires:
  3/1 -> out/1
  2/1 -> 3/2
  1/1 -> 3/1
  36/1 -> 2/2, 1/2
  in2/1 -> 2/1
  in1/1 -> 1/1

== system mylib/278_dzt_v1/diff_brake/calc_brake_Ib/cut_brake_4/z_ch1 ==
  in1 : Inport
  in2 : Inport  Port=2
  1 : RelationalOperator  Operator===  OutDataTypeStr=boolean  RndMeth=Simplest
  2 : RelationalOperator  Operator===  OutDataTypeStr=boolean  RndMeth=Simplest
  3 : Logic  AllPortsSameDT=off  OutDataTypeStr=boolean
  36 : Constant  Value=0
  out : Outport
  wires:
  3/1 -> out/1
  2/1 -> 3/2
  1/1 -> 3/1
  36/1 -> 2/2, 1/2
  in2/1 -> 2/1
  in1/1 -> 1/1

== system mylib/278_dzt_v1/diff_brake/calc_brake_Ib/cut_brake_4/z_ch2 ==
  in1 : Inport
  in2 : Inport  Port=2
  1 : RelationalOperator  Operator===  OutDataTypeStr=boolean  RndMeth=Simplest
  2 : RelationalOperator  Operator===  OutDataTypeStr=boolean  RndMeth=Simplest
  3 : Logic  AllPortsSameDT=off  OutDataTypeStr=boolean
  36 : Constant  Value=0
  out : Outport
  wires:
  3/1 -> out/1
  2/1 -> 3/2
  1/1 -> 3/1
  36/1 -> 2/2, 1/2
  in2/1 -> 2/1
  in1/1 -> 1/1

== system mylib/278_dzt_v1/diff_brake/calc_brake_Ic/cut_brake_1/ADD_B ==
  Y1 : Inport
  X2 : Inport  Port=2
  Y2 : Inport  Port=3
  X1 : Inport  Port=4
  1 : Product
  2 : Sum  Inputs=+-
  3 : Product  Inputs=*/  RndMeth=Zero  SaturateOnIntegerOverflow=on
  4 : Product
  5 : Sum  Inputs=+-
  out : Outport
  wires:
  3/1 -> out/1
  4/1 -> 5/2
  Y2/1 -> 4/1
  2/1 -> 3/2
  5/1 -> 3/1
  1/1 -> 5/1
  X2/1 -> 2/1, 1/2
  X1/1 -> 4/2, 2/2
  Y1/1 -> 1/1

== system mylib/278_dzt_v1/diff_brake/calc_brake_Ic/cut_brake_1/ADD_K ==
  Y2 : Inport
  Y1 : Inport  Port=2
  X2 : Inport  Port=3
  X1 : Inport  Port=4
  1 : Sum  Inputs=+-
  2 : Sum  Inputs=+-
  3 : Product  Inputs=*/  RndMeth=Zero  SaturateOnIntegerOverflow=on
  out : Outport
  wires:
  Y1/1 -> 1/2
  Y2/1 -> 1/1
  X1/1 -> 2/2
  X2/1 -> 2/1
  3/1 -> out/1
  2/1 -> 3/2
  1/1 -> 3/1

== system mylib/278_dzt_v1/diff_brake/calc_brake_Ic/cut_brake_1/z_ch ==
  in1 : Inport
  in2 : Inport  Port=2
  1 : RelationalOperator  Operator===  OutDataTypeStr=boolean  RndMeth=Simplest
  2 : RelationalOperator  Operator===  OutDataTypeStr=boolean  RndMeth=Simplest
  3 : Logic  AllPortsSameDT=off  OutDataTypeStr=boolean
  36 : Constant  Value=0
  out : Outport
  wires:
  3/1 -> out/1
  2/1 -> 3/2
  1/1 -> 3/1
  36/1 -> 2/2, 1/2
  in2/1 -> 2/1
  in1/1 -> 1/1

== system mylib/278_dzt_v1/diff_brake/calc_brake_Ic/cut_brake_1/z_ch1 ==
  in1 : Inport
  in2 : Inport  Port=2
  1 : RelationalOperator  Operator===  OutDataTypeStr=boolean  RndMeth=Simplest
  2 : RelationalOperator  Operator===  OutDataTypeStr=boolean  RndMeth=Simplest
  3 : Logic  AllPortsSameDT=off  OutDataTypeStr=boolean
  36 : Constant  Value=0
  out : Outport
  wires:
  3/1 -> out/1
  2/1 -> 3/2
  1/1 -> 3/1
  36/1 -> 2/2, 1/2
  in2/1 -> 2/1
  in1/1 -> 1/1

== system mylib/278_dzt_v1/diff_brake/calc_brake_Ic/cut_brake_1/z_ch2 ==
  in1 : Inport
  in2 : Inport  Port=2
  1 : RelationalOperator  Operator===  OutDataTypeStr=boolean  RndMeth=Simplest
  2 : RelationalOperator  Operator===  OutDataTypeStr=boolean  RndMeth=Simplest
  3 : Logic  AllPortsSameDT=off  OutDataTypeStr=boolean
  36 : Constant  Value=0
  out : Outport
  wires:
  3/1 -> out/1
  2/1 -> 3/2
  1/1 -> 3/1
  36/1 -> 2/2, 1/2
  in2/1 -> 2/1
  in1/1 -> 1/1

== system mylib/278_dzt_v1/diff_brake/calc_brake_Ic/cut_brake_2/ADD_B ==
  Y1 : Inport
  X2 : Inport  Port=2
  Y2 : Inport  Port=3
  X1 : Inport  Port=4
  1 : Product
  2 : Sum  Inputs=+-
  3 : Product  Inputs=*/  RndMeth=Zero  SaturateOnIntegerOverflow=on
  4 : Product
  5 : Sum  Inputs=+-
  out : Outport
  wires:
  3/1 -> out/1
  4/1 -> 5/2
  Y2/1 -> 4/1
  2/1 -> 3/2
  5/1 -> 3/1
  1/1 -> 5/1
  X2/1 -> 2/1, 1/2
  X1/1 -> 4/2, 2/2
  Y1/1 -> 1/1

== system mylib/278_dzt_v1/diff_brake/calc_brake_Ic/cut_brake_2/ADD_K ==
  Y2 : Inport
  Y1 : Inport  Port=2
  X2 : Inport  Port=3
  X1 : Inport  Port=4
  1 : Sum  Inputs=+-
  2 : Sum  Inputs=+-
  3 : Product  Inputs=*/  RndMeth=Zero  SaturateOnIntegerOverflow=on
  out : Outport
  wires:
  Y1/1 -> 1/2
  Y2/1 -> 1/1
  X1/1 -> 2/2
  X2/1 -> 2/1
  3/1 -> out/1
  2/1 -> 3/2
  1/1 -> 3/1

== system mylib/278_dzt_v1/diff_brake/calc_brake_Ic/cut_brake_2/z_ch ==
  in1 : Inport
  in2 : Inport  Port=2
  1 : RelationalOperator  Operator===  OutDataTypeStr=boolean  RndMeth=Simplest
  2 : RelationalOperator  Operator===  OutDataTypeStr=boolean  RndMeth=Simplest
  3 : Logic  AllPortsSameDT=off  OutDataTypeStr=boolean
  36 : Constant  Value=0
  out : Outport
  wires:
  3/1 -> out/1
  2/1 -> 3/2
  1/1 -> 3/1
  36/1 -> 2/2, 1/2
  in2/1 -> 2/1
  in1/1 -> 1/1

== system mylib/278_dzt_v1/diff_brake/calc_brake_Ic/cut_brake_2/z_ch1 ==
  in1 : Inport
  in2 : Inport  Port=2
  1 : RelationalOperator  Operator===  OutDataTypeStr=boolean  RndMeth=Simplest
  2 : RelationalOperator  Operator===  OutDataTypeStr=boolean  RndMeth=Simplest
  3 : Logic  AllPortsSameDT=off  OutDataTypeStr=boolean
  36 : Constant  Value=0
  out : Outport
  wires:
  3/1 -> out/1
  2/1 -> 3/2
  1/1 -> 3/1
  36/1 -> 2/2, 1/2
  in2/1 -> 2/1
  in1/1 -> 1/1

== system mylib/278_dzt_v1/diff_brake/calc_brake_Ic/cut_brake_2/z_ch2 ==
  in1 : Inport
  in2 : Inport  Port=2
  1 : RelationalOperator  Operator===  OutDataTypeStr=boolean  RndMeth=Simplest
  2 : RelationalOperator  Operator===  OutDataTypeStr=boolean  RndMeth=Simplest
  3 : Logic  AllPortsSameDT=off  OutDataTypeStr=boolean
  36 : Constant  Value=0
  out : Outport
  wires:
  3/1 -> out/1
  2/1 -> 3/2
  1/1 -> 3/1
  36/1 -> 2/2, 1/2
  in2/1 -> 2/1
  in1/1 -> 1/1

== system mylib/278_dzt_v1/diff_brake/calc_brake_Ic/cut_brake_3/ADD_B ==
  Y1 : Inport
  X2 : Inport  Port=2
  Y2 : Inport  Port=3
  X1 : Inport  Port=4
  1 : Product
  2 : Sum  Inputs=+-
  3 : Product  Inputs=*/  RndMeth=Zero  SaturateOnIntegerOverflow=on
  4 : Product
  5 : Sum  Inputs=+-
  out : Outport
  wires:
  3/1 -> out/1
  4/1 -> 5/2
  Y2/1 -> 4/1
  2/1 -> 3/2
  5/1 -> 3/1
  1/1 -> 5/1
  X2/1 -> 2/1, 1/2
  X1/1 -> 4/2, 2/2
  Y1/1 -> 1/1

== system mylib/278_dzt_v1/diff_brake/calc_brake_Ic/cut_brake_3/ADD_K ==
  Y2 : Inport
  Y1 : Inport  Port=2
  X2 : Inport  Port=3
  X1 : Inport  Port=4
  1 : Sum  Inputs=+-
  2 : Sum  Inputs=+-
  3 : Product  Inputs=*/  RndMeth=Zero  SaturateOnIntegerOverflow=on
  out : Outport
  wires:
  Y1/1 -> 1/2
  Y2/1 -> 1/1
  X1/1 -> 2/2
  X2/1 -> 2/1
  3/1 -> out/1
  2/1 -> 3/2
  1/1 -> 3/1

== system mylib/278_dzt_v1/diff_brake/calc_brake_Ic/cut_brake_3/z_ch ==
  in1 : Inport
  in2 : Inport  Port=2
  1 : RelationalOperator  Operator===  OutDataTypeStr=boolean  RndMeth=Simplest
  2 : RelationalOperator  Operator===  OutDataTypeStr=boolean  RndMeth=Simplest
  3 : Logic  AllPortsSameDT=off  OutDataTypeStr=boolean
  36 : Constant  Value=0
  out : Outport
  wires:
  3/1 -> out/1
  2/1 -> 3/2
  1/1 -> 3/1
  36/1 -> 2/2, 1/2
  in2/1 -> 2/1
  in1/1 -> 1/1

== system mylib/278_dzt_v1/diff_brake/calc_brake_Ic/cut_brake_3/z_ch1 ==
  in1 : Inport
  in2 : Inport  Port=2
  1 : RelationalOperator  Operator===  OutDataTypeStr=boolean  RndMeth=Simplest
  2 : RelationalOperator  Operator===  OutDataTypeStr=boolean  RndMeth=Simplest
  3 : Logic  AllPortsSameDT=off  OutDataTypeStr=boolean
  36 : Constant  Value=0
  out : Outport
  wires:
  3/1 -> out/1
  2/1 -> 3/2
  1/1 -> 3/1
  36/1 -> 2/2, 1/2
  in2/1 -> 2/1
  in1/1 -> 1/1

== system mylib/278_dzt_v1/diff_brake/calc_brake_Ic/cut_brake_3/z_ch2 ==
  in1 : Inport
  in2 : Inport  Port=2
  1 : RelationalOperator  Operator===  OutDataTypeStr=boolean  RndMeth=Simplest
  2 : RelationalOperator  Operator===  OutDataTypeStr=boolean  RndMeth=Simplest
  3 : Logic  AllPortsSameDT=off  OutDataTypeStr=boolean
  36 : Constant  Value=0
  out : Outport
  wires:
  3/1 -> out/1
  2/1 -> 3/2
  1/1 -> 3/1
  36/1 -> 2/2, 1/2
  in2/1 -> 2/1
  in1/1 -> 1/1

== system mylib/278_dzt_v1/diff_brake/calc_brake_Ic/cut_brake_4/ADD_B ==
  Y1 : Inport
  X2 : Inport  Port=2
  Y2 : Inport  Port=3
  X1 : Inport  Port=4
  1 : Product
  2 : Sum  Inputs=+-
  3 : Product  Inputs=*/  RndMeth=Zero  SaturateOnIntegerOverflow=on
  4 : Product
  5 : Sum  Inputs=+-
  out : Outport
  wires:
  3/1 -> out/1
  4/1 -> 5/2
  Y2/1 -> 4/1
  2/1 -> 3/2
  5/1 -> 3/1
  1/1 -> 5/1
  X2/1 -> 2/1, 1/2
  X1/1 -> 4/2, 2/2
  Y1/1 -> 1/1

== system mylib/278_dzt_v1/diff_brake/calc_brake_Ic/cut_brake_4/ADD_K ==
  Y2 : Inport
  Y1 : Inport  Port=2
  X2 : Inport  Port=3
  X1 : Inport  Port=4
  1 : Sum  Inputs=+-
  2 : Sum  Inputs=+-
  3 : Product  Inputs=*/  RndMeth=Zero  SaturateOnIntegerOverflow=on
  out : Outport
  wires:
  Y1/1 -> 1/2
  Y2/1 -> 1/1
  X1/1 -> 2/2
  X2/1 -> 2/1
  3/1 -> out/1
  2/1 -> 3/2
  1/1 -> 3/1
